simulink model "E1s"  (R2014a)
settings: Solver=ode45  StartTime=0.0  StopTime=1000  RelTol=1e-9
values from neighbouring files (symbols this model uses):
  Kr = 1    [E1.m]
libraries: cstblocks x3, simulink x2
settings Model: Creator=Davide  LastModifiedBy=Davide

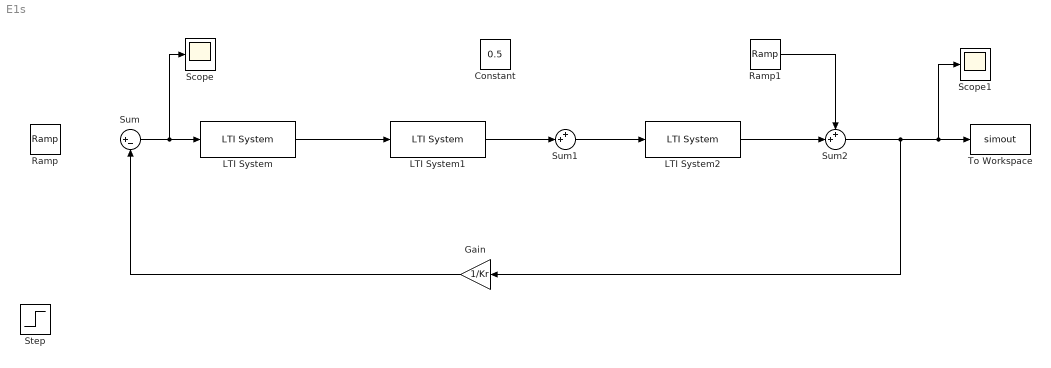
== system E1s ==
  Constant : Constant  Value=0.5
  Gain : Gain  Gain=1/Kr
  LTI System : cstblocks/LTI System  sys=C  IC=[]
  LTI System1 : cstblocks/LTI System  sys=F1  IC=[]
  LTI System2 : cstblocks/LTI System  sys=F2  IC=[]
  Ramp : simulink/Sources/Ramp  slope=1  start=0  X0=0
  Ramp1 : simulink/Sources/Ramp  slope=0.1  start=0  X0=0
  Scope : Scope
  Scope1 : Scope
  Step : Step  SampleTime=0
  Sum : Sum  Inputs=|+-
  Sum1 : Sum  Inputs=++|
  Sum2 : Sum  Inputs=++|
  To Workspace : ToWorkspace  VariableName=simout  SaveFormat=Timeseries  SampleTime=-1
  wires:
  Sum2/1 -> Gain/1, Scope1/1, To Workspace/1
  Gain/1 -> Sum/2
  Sum/1 -> Scope/1, LTI System/1
  LTI System/1 -> LTI System1/1
  LTI System1/1 -> Sum1/2
  Sum1/1 -> LTI System2/1
  LTI System2/1 -> Sum2/2
  Ramp1/1 -> Sum2/1
